simulink model "QPSK"  (R2018b)
settings: Solver=FixedStepAuto  StartTime=0.0  StopTime=1  FixedStep=1e-3  RelTol=1e-3
libraries: simulink x2, commdigbbndpm3 x1, commrandsrc3 x1
settings Model: Creator=marcone  LastModifiedBy=marcone

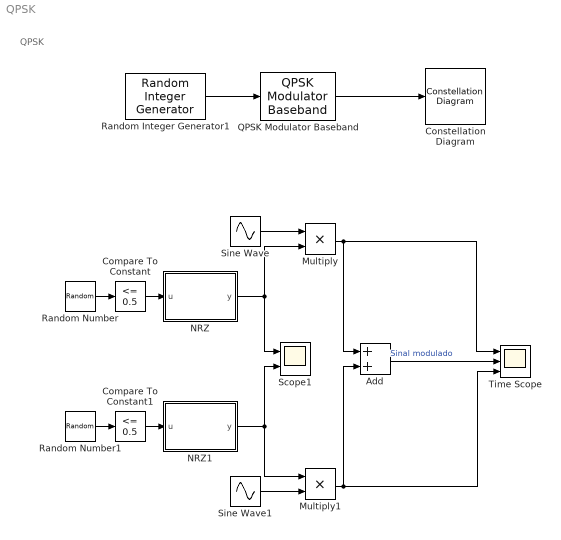
== system QPSK ==
  note: QPSK
  Add : Sum
  Compare To Constant : simulink/Logic and Bit Operations/Compare To Constant  relop=<=  const=0.5  OutDataTypeStr=boolean
  Compare To Constant1 : simulink/Logic and Bit Operations/Compare To Constant  relop=<=  const=0.5  OutDataTypeStr=boolean
  Constellation Diagram : ConstellationDiagram
  Multiply : Product
  Multiply1 : Product
  NRZ : MATLAB Function  TreatAsAtomicUnit=on
  NRZ1 : MATLAB Function  TreatAsAtomicUnit=on
  QPSK Modulator Baseband : commdigbbndpm3/QPSK Modulator Baseband  InType=Integer  Enc=Gray  Ph=pi/4  outDtype=double  outWordLen=16  outUDDataType=sfix(16)  outFracLenMode=Best precision  outFracLen=15  outDataTypeStr=double  outLastDataTypeStr=double
  Random Number : RandomNumber  Mean=0.5  SampleTime=0.1
  Random Number1 : RandomNumber  Mean=0.5  Seed=10  SampleTime=0.1
  Random Integer Generator1 : commrandsrc3/Random Integer Generator  SetSize=4  SeedSource=Auto  Seed=0  SampleTime=1  SamplesPerFrame=10000  OutputDataType=double  SimulateUsing=Interpreted execution
  Scope1 : Scope  NumInputPorts=2
  Sine Wave : Sin  Amplitude=2  Frequency=500  SampleTime=0
  Sine Wave1 : Sin  Amplitude=2  Frequency=500  Phase=90*pi/180  SampleTime=0
  Time Scope : Scope  NumInputPorts=3
  wires:
  Random Integer Generator1/1 -> QPSK Modulator Baseband/1
  Compare To Constant/1 -> NRZ/1(u)
  Compare To Constant1/1 -> NRZ1/1(u)
  NRZ/1(y) -> Multiply/2, Scope1/1
  NRZ1/1(y) -> Multiply1/1, Scope1/2
  Random Number/1 -> Compare To Constant/1
  Random Number1/1 -> Compare To Constant1/1
  Sine Wave/1 -> Multiply/1
  Multiply/1 -> Time Scope/1, Add/1
  Multiply1/1 -> Time Scope/3, Add/2
  Sine Wave1/1 -> Multiply1/2
  Add/1 -> Time Scope/2  "Sinal modulado"
  QPSK Modulator Baseband/1 -> Constellation Diagram/1

== matlab function QPSK/NRZ1 ==
  data: u input; y output
function y = fcn(u)
if u == 1
    y = 1;
else
    y = -1;
end
end

== matlab function QPSK/NRZ ==
  data: u input; y output
function y = fcn(u)
if u == 1
    y = 1;
else
    y = -1;
end
end
